simulink subsystem "getIonoPiercePoint"  (R2021a)
settings: Solver=VariableStepAuto  StartTime=0.0  StopTime=10.0  RelTol=1e-3
undefined symbols (not defined in the file): IPP_RefAltitude, Re
settings Model: Creator=zurnmar  LastModifiedBy=zurnmar

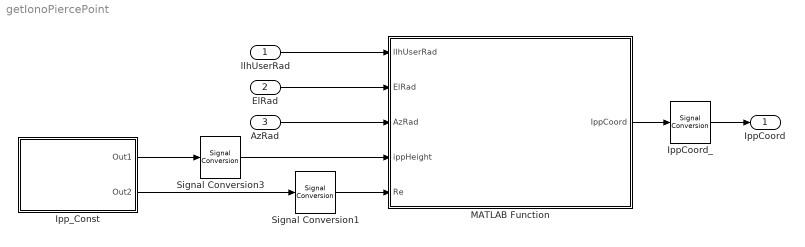
== system getIonoPiercePoint ==
  llhUserRad : Inport
  ElRad : Inport  Port=2
  AzRad : Inport  Port=3
  IppCoord_ : SignalConversion  OverrideOpt=off
  Ipp_Const : Subsystem
  MATLAB Function : MATLAB Function  TreatAsAtomicUnit=on
  Signal Conversion1 : SignalConversion  OverrideOpt=off
  Signal Conversion3 : SignalConversion  OverrideOpt=off
  IppCoord : Outport
  wires:
  llhUserRad/1 -> MATLAB Function/1(llhUserRad)
  MATLAB Function/1(IppCoord) -> IppCoord_/1
  AzRad/1 -> MATLAB Function/3(AzRad)
  Ipp_Const/1(Out1) -> Signal Conversion3/1
  ElRad/1 -> MATLAB Function/2(ElRad)
  Signal Conversion3/1 -> MATLAB Function/4(ippHeight)
  IppCoord_/1 -> IppCoord/1
  Signal Conversion1/1 -> MATLAB Function/5(Re)
  Ipp_Const/2(Out2) -> Signal Conversion1/1

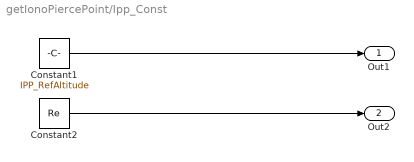
== system getIonoPiercePoint/Ipp_Const ==
  Constant1 : Constant  Value=IPP_RefAltitude
  Constant2 : Constant  Value=Re
  Out1 : Outport
  Out2 : Outport  Port=2
  wires:
  Constant2/1 -> Out2/1
  Constant1/1 -> Out1/1

== matlab function getIonoPiercePoint/MATLAB Function ==
  data: llhUserRad input; IppCoord output; ElRad input; AzRad input; ippHeight input; Re input
% *************************************************************************
% Point of intersection between the line joining receiver and satellite
% positions and the imaginary thin ionospheric shell at ippHeight (typically 450 km or 350 km)
% llhUserRad is receiver's position in LLH [rad]%
% ElRad is satellite elevation [rad]
% AzRad is satellite azimuth [rad]
% ippHeight is the height of the imaginary thin ionospheric shell
% *************************************************************************
function IppCoord  = getIonoPiercePoint(llhUserRad,ElRad,AzRad,ippHeight,Re)
IppCoord=[0;0];

if isempty(ippHeight)
    h_IPP = 450*1e3; % or 350*1e3
else    
    h_IPP = ippHeight; % or 350*1e3
end
r = h_IPP+Re;

Psi_pp    = pi/2 - ElRad - asin(Re/r.*cos(ElRad));
sinPsi_pp = sin(Psi_pp);
IppCoord(1,1) = (asin(sin(llhUserRad(1,1)).*cos(Psi_pp)+cos(llhUserRad(1,1)).*sinPsi_pp.*cos(AzRad)));
IppCoord(2,1) = (llhUserRad(2,1) + asin(sinPsi_pp.*sin(AzRad)./cos(IppCoord(1,1))));
